simulink model "CertPendLinear"  (R2017a)
settings: Solver=VariableStepAuto  StartTime=0.0  StopTime=1  RelTol=1e-3
values from neighbouring files (symbols this model uses):
  b = 0.1    [CartParams.m]
  g = 10    [CartParams.m]
  I = 0.006    [CartParams.m]
  l = 0.3    [CartParams.m]
  m = 0.2    [CartParams.m]
  M = 0.5    [CartParams.m]
settings Model: Creator=hkariti  LastModifiedBy=hkariti

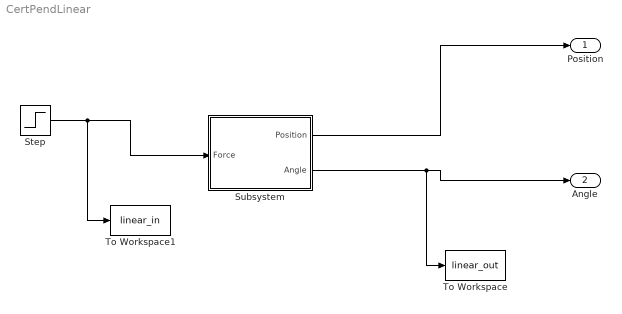
== system CertPendLinear ==
  Step : Step  Time=0  SampleTime=0
  Subsystem : Subsystem
  To Workspace : ToWorkspace  VariableName=linear_out  SaveFormat=Timeseries  SampleTime=-1
  To Workspace1 : ToWorkspace  VariableName=linear_in  SaveFormat=Timeseries  SampleTime=-1
  Position : Outport
  Angle : Outport  Port=2
  wires:
  Step/1 -> To Workspace1/1, Subsystem/1(Force)
  Subsystem/1(Position) -> Position/1
  Subsystem/2(Angle) -> To Workspace/1, Angle/1

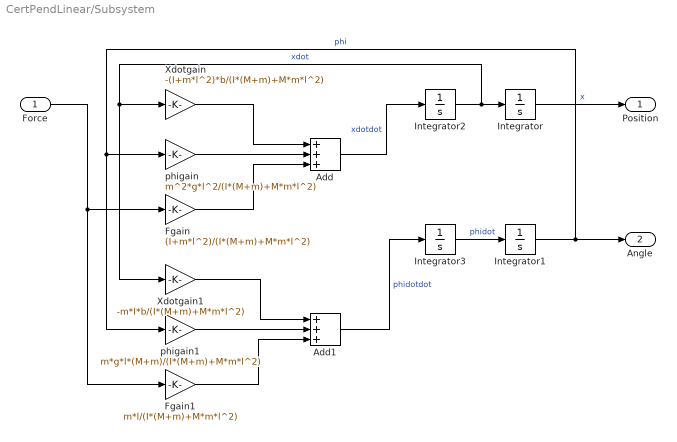
== system CertPendLinear/Subsystem ==
  Force : Inport
  Add : Sum  Inputs=+++
  Add1 : Sum  Inputs=+++
  Fgain : Gain  Gain=(I+m*l^2)/(I*(M+m)+M*m*l^2)
  Fgain1 : Gain  Gain=m*l/(I*(M+m)+M*m*l^2)
  Integrator{,1..3} (4 alike) : Integrator
  Xdotgain : Gain  Gain=-(I+m*l^2)*b/(I*(M+m)+M*m*l^2)
  Xdotgain1 : Gain  Gain=-m*l*b/(I*(M+m)+M*m*l^2)
  phigain : Gain  Gain=m^2*g*l^2/(I*(M+m)+M*m*l^2)
  phigain1 : Gain  Gain=m*g*l*(M+m)/(I*(M+m)+M*m*l^2)
  Position : Outport
  Angle : Outport  Port=2
  wires:
  Fgain/1 -> Add/3
  Fgain1/1 -> Add1/3
  Add1/1 -> Integrator3/1  "phidotdot"
  Xdotgain1/1 -> Add1/1
  phigain/1 -> Add/2
  Integrator/1 -> Position/1  "x"
  Integrator1/1 -> Angle/1, phigain/1, phigain1/1  "phi"
  Integrator2/1 -> Xdotgain1/1, Xdotgain/1, Integrator/1  "xdot"
  Force/1 -> Fgain1/1, Fgain/1
  Xdotgain/1 -> Add/1
  Integrator3/1 -> Integrator1/1  "phidot"
  phigain1/1 -> Add1/2
  Add/1 -> Integrator2/1  "xdotdot"
